simulink model "battery"  (R2021a)
settings: Solver=ode3  StartTime=0.0  StopTime=inf  FixedStep=T_est  RelTol=1e-3  EnableMultiTasking=on
values from neighbouring files (symbols this model uses):
  C1_array = [10000 10000 20775.14128 59367.58362 2271.12322 25499.34704 24626.77363 22758.69305 1470.76099 16269.06063 343.94923 166277.12244 ... (44 elements, 11x4)]    [ecmparams_vsc.mat]    (also in load_sim_data.m = [ecmparams(1:3,2)'; ecmparams(4:6,2)'; ecmparams(7:9,2)']; load_sim_data_v2.m = [ecmparams(1:3,2)'; ecmparams(4:6,2)'; ecmparams(7:9,2)'])
  C2_array = [5000 5000 3386.51997 1284.26954 733.57385 21.9068258 408.44714 1025.29527 23.88432 4732.43934 4.98786 7213.94612 ... (44 elements, 11x4)]    [ecmparams_vsc.mat]    (also in load_sim_data.m = [ecmparams(1:3,4)'; ecmparams(4:6,4)'; ecmparams(7:9,4)']; load_sim_data_v2.m = [ecmparams(1:3,4)'; ecmparams(4:6,4)'; ecmparams(7:9,4)'])
  cell_soc_init = initial_soc*ones(ns,nl,nc)    [load_sim_data.m]
  cell_temp = 25*ones(ns,nl,nc)    [load_sim_data.m]
  drive_profile = [0.003069801 0.003247245 0.003020715 0.003053892 0.002820143 0.003317081 0.003158873 0.002919445 0.002956375 0.002698265 0.002861501 0.002770798 ... (18750 elements, 1x18750)]    [drive_profile_ftp.mat]    (also in workspace.mat = [0 0 0 0 0 0 0 0 0 0 0 0 ... (521 elements, 1x521)]; workspace_2rc.mat; workspace_comparison.mat)
  drive_profile_index = [1 2 3 4 5 6 7 8 9 10 11 12 ... (18750 elements, 1x18750)]    [drive_profile_ftp.mat]    (also in load_sim_data_v2.m = drive_profile_index - 1; workspace.mat = [0 0.115384615385 0.230769230769 0.346153846154 0.4615384615; workspace_2rc.mat; workspace_comparison.mat)
  initial_soc = interp1(voc_soc_lut, voc_soc_lut_index, initial_vterm)    [load_sim_data.m]    (also in load_sim_data_v2.m)
  initial_temp = 25    [load_sim_data.m]    (also in load_sim_data_v2.m)
  nc = 1    [load_sim_data.m]
  nl = 1    [load_sim_data.m]
  nm = 1    [load_sim_data.m]
  ns = 1    [load_sim_data.m]
  Q_total = 236.8    [load_sim_data.m]    (also in load_sim_data_v2.m = 350; workspace.mat = 44; workspace_2rc.mat = 44; workspace_comparison.mat = 44)
  R1 = interp2(temp_array, voc_array, R1_array, initial_temp, initial_voc)    [load_sim_data.m]    (also in load_sim_data_v2.m; workspace.mat = 0.00033425; workspace_2rc.mat = 0.0001483; workspace_comparison.mat = 0.0001483)
  R1_array = [0.001 0.001 0.00171 0.00621 0.00621 0.00495 0.00657 0.00419 0.01404 0.0095 0.00356 0.01783 ... (44 elements, 11x4)]    [ecmparams_vsc.mat]    (also in load_sim_data.m = [ecmparams(1:3,3)'; ecmparams(4:6,3)'; ecmparams(7:9,3)']; load_sim_data_v2.m = [ecmparams(1:3,3)'; ecmparams(4:6,3)'; ecmparams(7:9,3)'])
  R2 = interp2(temp_array, voc_array, R2_array, initial_temp, initial_voc)    [load_sim_data.m]    (also in load_sim_data_v2.m; workspace.mat = 0.000915125; workspace_2rc.mat = 0.0001594; workspace_comparison.mat = 0.0001594)
  R2_array = [0.001 0.001 0.00067 0.01044 0.00794 0.01181 0.0098 0.00694 0.00323 0.00236 0.02009 0.00195 ... (44 elements, 11x4)]    [ecmparams_vsc.mat]    (also in load_sim_data.m = [ecmparams(1:3,5)'; ecmparams(4:6,5)'; ecmparams(7:9,5)']; load_sim_data_v2.m = [ecmparams(1:3,5)'; ecmparams(4:6,5)'; ecmparams(7:9,5)'])
  Ri = interp2(temp_array, voc_array, Ri_array, initial_temp, initial_voc)    [load_sim_data.m]    (also in load_sim_data_v2.m; workspace.mat = 0.000736040625; workspace_2rc.mat = 0.0007932; workspace_comparison.mat = 0.0007932)
  Ri_array = [0.001 0.001 0.00089 0.02157 0.01286 0.00303 0.0054 0.0079 0.00204 0.01221 0.00632 0.00315 ... (44 elements, 11x4)]    [ecmparams_vsc.mat]    (also in load_sim_data.m = [ecmparams(1:3,1)'; ecmparams(4:6,1)'; ecmparams(7:9,1)']; load_sim_data_v2.m = [ecmparams(1:3,1)'; ecmparams(4:6,1)'; ecmparams(7:9,1)'])
  sim_time = drive_profile_index(end)    [load_sim_data.m]    (also in load_sim_data_v2.m)
  temp_array = [15 25 35]    [load_sim_data.m]    (also in load_sim_data_v2.m)
  voc_array = [3 3.6 4.2]    [load_sim_data.m]    (also in load_sim_data_v2.m)
  voc_soc_lut = [3.07420931 3.44278771 3.51037487 3.58546258 3.63776945 3.68066188 3.73931818 3.84140797 3.94332291 4.0535654 4.18301283]    [emf_curve_single.mat]    (also in workspace.mat = [2.9985 3.0047 3.1504 3.2397 3.3026 3.3438 3.3699 3.3878 3.4; workspace_2rc.mat = [2.9985 3.0047 3.1504 3.2397 3.3026 3.3438 3.3699 3.3878 3.4; workspace_comparison.mat = [2.9985 3.0047 3.1504 3.2397 3.3026 3.3438 3.3699 3.3878 3.4)
  voc_soc_lut_index = [0 10 20 30 40 50 60 70 80 90 100]    [emf_curve_single.mat]    (also in workspace.mat = [0 1.6393442623 3.27868852459 4.91803278689 6.55737704918 8.; workspace_2rc.mat = [0 1.6393442623 3.27868852459 4.91803278689 6.55737704918 8.; workspace_comparison.mat = [0 1.6393442623 3.27868852459 4.91803278689 6.55737704918 8.)
undefined symbols (not defined in the file or in its folder): cell_c1_init, cell_c2_init, cell_r0_init, cell_r1_init, cell_r2_init
libraries: fl_lib x17, nesl_utility x11
settings Model: Creator=OTG00077  LastModifiedBy=avramkachura
settings SolverCC: AlgebraicLoopSolver=TrustRegion
settings DataIOCC: LimitDataPoints=on  SaveFormat=Array  ReturnWorkspaceOutputs=off
settings OptimizationCC: LifeSpan=inf
settings DebuggingCC: SolverPrmCheckMsg=warning  SFUnexpectedBacktrackingDiag=warning  SFNoUnconditionalDefaultTransitionDiag=warning  SFExecutionAtInitializationDiag=none  SFMachineParentedDataDiag=warning  ArithmeticOperatorsInVariantConditions=warning
settings HardwareCC: ProdBitPerPointer=32  ProdBitPerSizeT=32  ProdBitPerPtrDiffT=32  ProdLargestAtomicFloat=None  ProdIntDivRoundTo=Undefined  ProdEndianess=Unspecified  ProdWordSize=32  ProdHWDeviceType=32-bit Generic
settings ModelReferenceCC: PropagateSignalLabelsOutOfModel=off
settings SFSimCC: SimUseLocalCustomCode=off  CustomCodeUndefinedFunction=UseInterfaceOnly
settings RTWCC: RTWUseLocalCustomCode=off
settings CodeAppCC: StateflowObjectComments=on
settings GRTTargetCC: TargetLangStandard=C89/C90 (ANSI)
settings ConfigComp: CovMetricSettings=dw  CovSaveCumulativeToWorkspaceVar=on  CovSaveSingleToWorkspaceVar=on  CovExternalEMLEnable=off  CovSFcnEnable=off
settings SimscapeCC: SimscapeNormalizeSystem=off

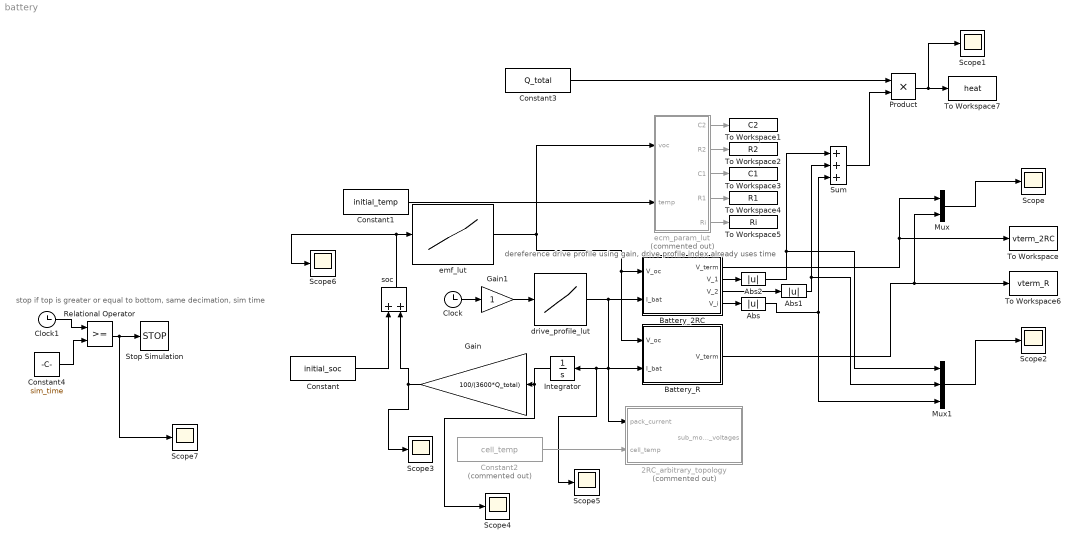
== system battery ==
  note: stop if top is greater or equal to bottom, same decimation, sim time
  note: dereference drive profile using gain, drive profile index already uses time
  2RC_arbitrary_topology : Subsystem  Commented=on
  Abs : Abs
  Abs1 : Abs
  Abs2 : Abs
  Battery_2RC : Subsystem
  Battery_R : Subsystem
  Clock : Clock
      settings: Decimation=100
  Clock1 : Clock
      settings: Decimation=100
  Constant : Constant  Value=initial_soc
  Constant1 : Constant  Value=initial_temp
  Constant2 : Constant  Commented=on  Value=cell_temp
  Constant3 : Constant  Value=Q_total
  Constant4 : Constant  Value=sim_time
  Gain : Gain  Gain=100/(3600*Q_total)
  Gain1 : Gain
  Integrator : Integrator
  Mux : Mux  Inputs=2
  Mux1 : Mux  Inputs=3
  Product : Product
  Relational Operator : RelationalOperator  OutDataTypeStr=boolean  RndMeth=Simplest
  Scope{,1..7} (8 alike) : Scope
  Stop Simulation : Stop
  Sum : Sum  Inputs=+++
  To Workspace : ToWorkspace  VariableName=vterm_2RC  SampleTime=-1
      settings: Decimation=100
  To Workspace1 : ToWorkspace  VariableName=C2  SampleTime=-1
      settings: MaxDataPoints=1  Decimation=100
  To Workspace2 : ToWorkspace  VariableName=R2  SampleTime=-1
      settings: MaxDataPoints=1  Decimation=100
  To Workspace3 : ToWorkspace  VariableName=C1  SampleTime=-1
      settings: MaxDataPoints=1  Decimation=100
  To Workspace4 : ToWorkspace  VariableName=R1  SampleTime=-1
      settings: MaxDataPoints=1  Decimation=100
  To Workspace5 : ToWorkspace  VariableName=Ri  SampleTime=-1
      settings: MaxDataPoints=1  Decimation=100
  To Workspace6 : ToWorkspace  VariableName=vterm_R  SampleTime=-1
      settings: Decimation=100
  To Workspace7 : ToWorkspace  VariableName=heat  SampleTime=-1
      settings: Decimation=100
  drive_profile_lut : Lookup_n-D  NumberOfTableDimensions=1  BreakpointsForDimension1=drive_profile_index  Table=drive_profile  InternalRulePriority=Speed  RndMeth=Simplest  InputSameDT=on
  "ecm_param_lut " : Subsystem  Commented=on
  emf_lut : Lookup_n-D  NumberOfTableDimensions=1  BreakpointsForDimension1=voc_soc_lut_index  Table=voc_soc_lut  InternalRulePriority=Speed  RndMeth=Simplest  InputSameDT=on
  soc : Sum
  wires:
  Integrator/1 -> Scope4/1, Gain/1
  Gain/1 -> Scope3/1, soc/2
  soc/1 -> Scope6/1, emf_lut/1
  Constant/1 -> soc/1
  emf_lut/1 -> "ecm_param_lut "/1(voc), Battery_R/1(V_oc), Battery_2RC/1(V_oc)
  drive_profile_lut/1 -> Battery_2RC/2(I_bat), Scope5/1, Integrator/1, 2RC_arbitrary_topology/1(pack_current), Battery_R/2(I_bat)
  Battery_2RC/1(V_term) -> Mux/1, To Workspace/1
  Clock/1 -> Gain1/1
  Gain1/1 -> drive_profile_lut/1
  Mux/1 -> Scope/1
  Battery_R/1(V_term) -> Mux/2, To Workspace6/1
  "ecm_param_lut "/1(C2) -> To Workspace1/1
  "ecm_param_lut "/2(R2) -> To Workspace2/1
  "ecm_param_lut "/5(Ri) -> To Workspace5/1
  "ecm_param_lut "/4(R1) -> To Workspace4/1
  "ecm_param_lut "/3(C1) -> To Workspace3/1
  Constant1/1 -> "ecm_param_lut "/2(temp)
  Constant2/1 -> 2RC_arbitrary_topology/2(cell_temp)
  Product/1 -> Scope1/1, To Workspace7/1
  Sum/1 -> Product/2
  Constant3/1 -> Product/1
  Battery_2RC/4(V_i) -> Abs/1
  Battery_2RC/3(V_2) -> Abs1/1
  Battery_2RC/2(V_1) -> Abs2/1
  Abs2/1 -> Mux1/1, Sum/1
  Abs1/1 -> Mux1/2, Sum/2
  Abs/1 -> Sum/3, Mux1/3
  Mux1/1 -> Scope2/1
  Relational Operator/1 -> Scope7/1, Stop Simulation/1
  Constant4/1 -> Relational Operator/2
  Clock1/1 -> Relational Operator/1

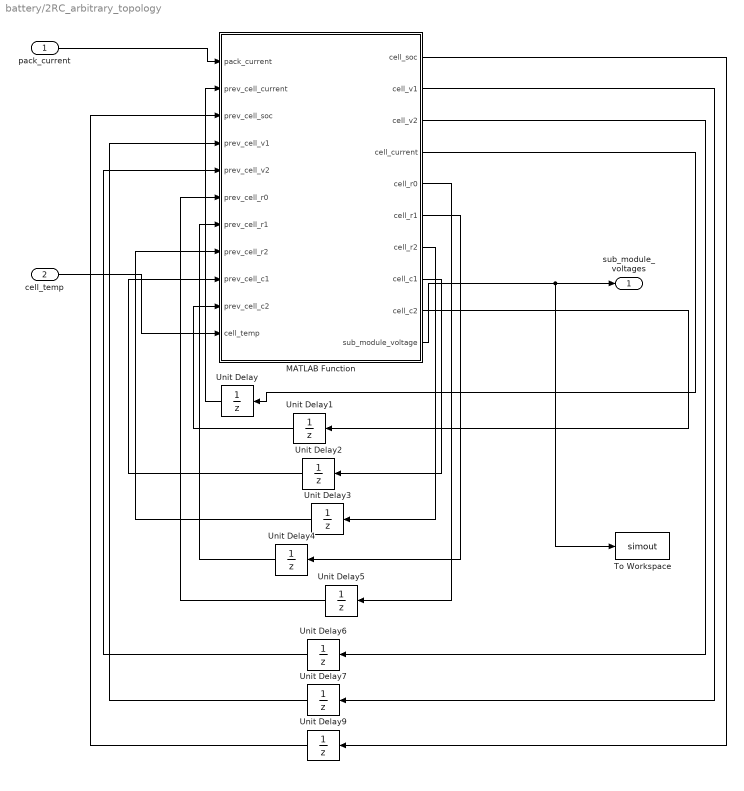
== system battery/2RC_arbitrary_topology ==
  pack_current : Inport
  cell_temp : Inport  Port=2
  MATLAB Function : MATLAB Function  TreatAsAtomicUnit=on
  To Workspace : ToWorkspace  VariableName=simout  SaveFormat=Timeseries  SampleTime=-1
  Unit Delay : UnitDelay  SampleTime=-1  HasFrameUpgradeWarning=on
  Unit Delay1 : UnitDelay  InitialCondition=cell_c2_init  SampleTime=-1  HasFrameUpgradeWarning=on
  Unit Delay2 : UnitDelay  InitialCondition=cell_c1_init  SampleTime=-1  HasFrameUpgradeWarning=on
  Unit Delay3 : UnitDelay  InitialCondition=cell_r2_init  SampleTime=-1  HasFrameUpgradeWarning=on
  Unit Delay4 : UnitDelay  InitialCondition=cell_r1_init  SampleTime=-1  HasFrameUpgradeWarning=on
  Unit Delay5 : UnitDelay  InitialCondition=cell_r0_init  SampleTime=-1  HasFrameUpgradeWarning=on
  Unit Delay6 : UnitDelay  SampleTime=-1  HasFrameUpgradeWarning=on
  Unit Delay7 : UnitDelay  SampleTime=-1  HasFrameUpgradeWarning=on
  Unit Delay9 : UnitDelay  InitialCondition=cell_soc_init  SampleTime=-1  HasFrameUpgradeWarning=on
  sub_module_voltages : Outport  VectorParamsAs1DForOutWhenUnconnected=off
  wires:
  pack_current/1 -> MATLAB Function/1(pack_current)
  cell_temp/1 -> MATLAB Function/11(cell_temp)
  MATLAB Function/10(sub_module_voltage) -> To Workspace/1, sub_module_voltages/1
  MATLAB Function/9(cell_c2) -> Unit Delay1/1
  Unit Delay1/1 -> MATLAB Function/10(prev_cell_c2)
  MATLAB Function/8(cell_c1) -> Unit Delay2/1
  Unit Delay2/1 -> MATLAB Function/9(prev_cell_c1)
  MATLAB Function/7(cell_r2) -> Unit Delay3/1
  Unit Delay3/1 -> MATLAB Function/8(prev_cell_r2)
  MATLAB Function/6(cell_r1) -> Unit Delay4/1
  Unit Delay4/1 -> MATLAB Function/7(prev_cell_r1)
  MATLAB Function/5(cell_r0) -> Unit Delay5/1
  Unit Delay5/1 -> MATLAB Function/6(prev_cell_r0)
  MATLAB Function/3(cell_v2) -> Unit Delay6/1
  Unit Delay6/1 -> MATLAB Function/5(prev_cell_v2)
  MATLAB Function/2(cell_v1) -> Unit Delay7/1
  Unit Delay7/1 -> MATLAB Function/4(prev_cell_v1)
  Unit Delay9/1 -> MATLAB Function/3(prev_cell_soc)
  MATLAB Function/4(cell_current) -> Unit Delay/1
  Unit Delay/1 -> MATLAB Function/2(prev_cell_current)
  MATLAB Function/1(cell_soc) -> Unit Delay9/1

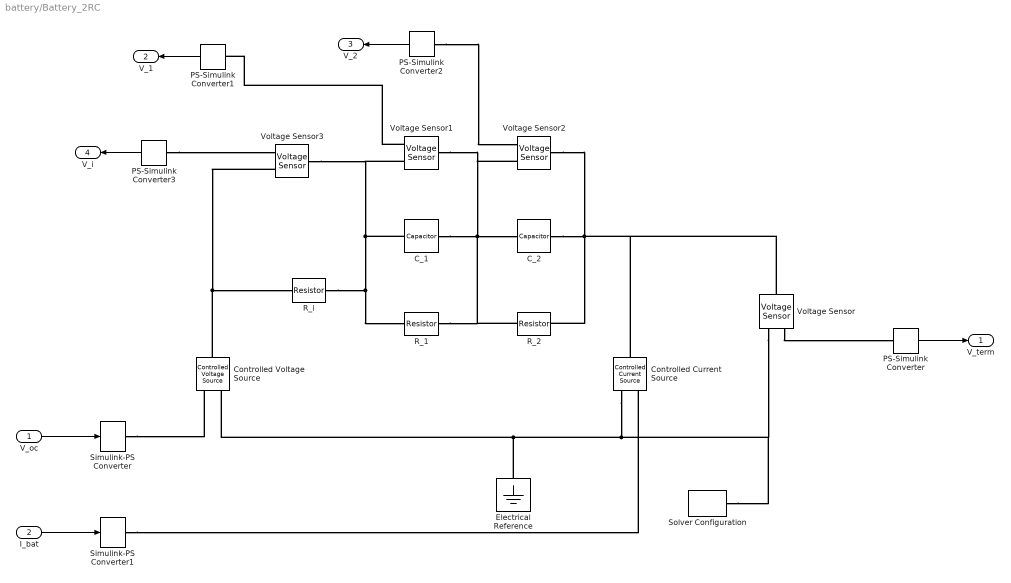
== system battery/Battery_2RC ==
  V_oc : Inport
  I_bat : Inport  Port=2
  C_1 : fl_lib/Electrical/Electrical Elements/Capacitor  c=C1 F  r=0 Ohm  g=0 1/Ohm  i_specify=off  i_priority=High  i=0 A  i_nominal_specify=off  i_nominal_unit=A  i_nominal_value=1  v_specify=off  v_priority=High  v=0 V  v_nominal_specify=off  v_nominal_unit=V  v_nominal_value=1  vc_specify=off  vc_priority=High  vc=0 V  vc_nominal_specify=off  vc_nominal_unit=V  vc_nominal_value=1
  C_2 : fl_lib/Electrical/Electrical Elements/Capacitor  c=C2 F  r=0 Ohm  g=0 1/Ohm  i_specify=off  i_priority=High  i=0 A  i_nominal_specify=off  i_nominal_unit=A  i_nominal_value=1  v_specify=off  v_priority=High  v=0 V  v_nominal_specify=off  v_nominal_unit=V  v_nominal_value=1  vc_specify=off  vc_priority=High  vc=0 V  vc_nominal_specify=off  vc_nominal_unit=V  vc_nominal_value=1
  Controlled Current Source : fl_lib/Electrical/Electrical Sources/Controlled Current Source
  Controlled Voltage Source : fl_lib/Electrical/Electrical Sources/Controlled Voltage Source
  Electrical Reference : fl_lib/Electrical/Electrical Elements/Electrical Reference
  PS-Simulink Converter{,1..3} (4 alike) : nesl_utility/PS-Simulink Converter  PhysicalDomain=network_engine_domain  SubClassName=ps_output  LeftPortType=input  RightPortType=output  PseudoPeriodic=off  Frequencies=[]  Unit=1  AffineConversion=off
      settings: SourceProductBaseCode=PW,SS
  R_1 : fl_lib/Electrical/Electrical Elements/Resistor  R=R1 Ohm  i_specify=off  i_priority=High  i=0 A  i_nominal_specify=off  i_nominal_unit=A  i_nominal_value=1  v_specify=off  v_priority=High  v=0 V  v_nominal_specify=off  v_nominal_unit=V  v_nominal_value=1
  R_2 : fl_lib/Electrical/Electrical Elements/Resistor  R=R2 Ohm  i_specify=off  i_priority=High  i=0 A  i_nominal_specify=off  i_nominal_unit=A  i_nominal_value=1  v_specify=off  v_priority=High  v=0 V  v_nominal_specify=off  v_nominal_unit=V  v_nominal_value=1
  R_i : fl_lib/Electrical/Electrical Elements/Resistor  R=Ri Ohm  i_specify=off  i_priority=High  i=0 A  i_nominal_specify=off  i_nominal_unit=A  i_nominal_value=1  v_specify=off  v_priority=High  v=0 V  v_nominal_specify=off  v_nominal_unit=V  v_nominal_value=1
  Simulink-PS Converter : nesl_utility/Simulink-PS Converter  PhysicalDomain=network_engine_domain  SubClassName=ps_input  LeftPortType=input  RightPortType=output  PseudoPeriodic=off  Frequencies=[]  NoiseDistribution=none  NoiseParameters=[]  Unit=1  AffineConversion=off  FilteringAndDerivatives=zero  SimscapeFilterOrder=1  InputFilterTimeConstant=0.001  UdotUserProvided=1
      settings: SourceProductBaseCode=PW,SS
  Simulink-PS Converter1 : nesl_utility/Simulink-PS Converter  PhysicalDomain=network_engine_domain  SubClassName=ps_input  LeftPortType=input  RightPortType=output  PseudoPeriodic=off  Frequencies=[]  NoiseDistribution=none  NoiseParameters=[]  Unit=1  AffineConversion=off  FilteringAndDerivatives=zero  SimscapeFilterOrder=1  InputFilterTimeConstant=0.001  UdotUserProvided=1
      settings: SourceProductBaseCode=PW,SS
  Solver Configuration : nesl_utility/Solver Configuration  PhysicalDomain=network_engine_domain  SubClassName=solver  LeftPortType=input  RightPortType=generic  Tones=[]  Harmonics=[]  SimulateNoise=off  Profile=off  UseLocalSampling=off  EnableSwitchedLinearOptims=on  FrequencyDomain=off  UseCCode=off  RelTol=0.001  AbsTol=1e-06  MinStep=1e-09  ToWorkspace=off  RevertToSquareIcSolve=off  NumHomotopyIterations=100  PhasorMode=off  PhasorModeNumHarmonics=1  DoDC=off  ResidualTolerance=1e-09  UseLocalSolver=off  LocalSolverChoice=NE_BACKWARD_EULER_ADVANCER  LocalSolverSampleTime=0.001  DoFixedCost=off  MaxNonlinIter=3  MaxModeIter=2  ComputeImpulses=off  ImpulseIterations=2  LinearAlgebra=Sparse  EquationFormulation=NE_TIME_EF  DelaysMemoryBudget=1024  AutomaticFiltering=on  FilteringTimeConstant=0.001  PartitionStorageMethod=AS_NEEDED  PartitionMemoryBudget=1024  PartitionMethod=FAST
      settings: SourceProductBaseCode=PW,SS
  Voltage Sensor{,1..3} (4 alike) : fl_lib/Electrical/Electrical Sensors/Voltage Sensor
  V_term : Outport  VectorParamsAs1DForOutWhenUnconnected=off
  V_1 : Outport  Port=2  VectorParamsAs1DForOutWhenUnconnected=off
  V_2 : Outport  Port=3  VectorParamsAs1DForOutWhenUnconnected=off
  V_i : Outport  Port=4  VectorParamsAs1DForOutWhenUnconnected=off
  wires:
  V_oc/1 -> Simulink-PS Converter/1
  PS-Simulink Converter/1 -> V_term/1
  I_bat/1 -> Simulink-PS Converter1/1
  PS-Simulink Converter1/1 -> V_1/1
  PS-Simulink Converter2/1 -> V_2/1
  PS-Simulink Converter3/1 -> V_i/1
  connections:
  R_i/RConn1 -- Voltage Sensor3/LConn1 -- Voltage Sensor1/RConn2 -- C_1/LConn1 -- R_1/LConn1
  C_1/RConn1 -- Voltage Sensor2/RConn2 -- Voltage Sensor1/LConn1 -- R_2/LConn1 -- R_1/RConn1 -- C_2/LConn1
  C_2/RConn1 -- Voltage Sensor2/LConn1 -- R_2/RConn1 -- Controlled Current Source/LConn1 -- Voltage Sensor/LConn1
  Controlled Voltage Source/LConn1 -- Voltage Sensor3/RConn2 -- R_i/LConn1
  Simulink-PS Converter/RConn1 -- Controlled Voltage Source/RConn1
  Voltage Sensor/RConn1 -- PS-Simulink Converter/LConn1
  Controlled Current Source/RConn2 -- Solver Configuration/RConn1 -- Voltage Sensor/RConn2 -- Electrical Reference/LConn1 -- Controlled Voltage Source/RConn2
  Simulink-PS Converter1/RConn1 -- Controlled Current Source/RConn1
  Voltage Sensor1/RConn1 -- PS-Simulink Converter1/LConn1
  PS-Simulink Converter2/LConn1 -- Voltage Sensor2/RConn1
  PS-Simulink Converter3/LConn1 -- Voltage Sensor3/RConn1

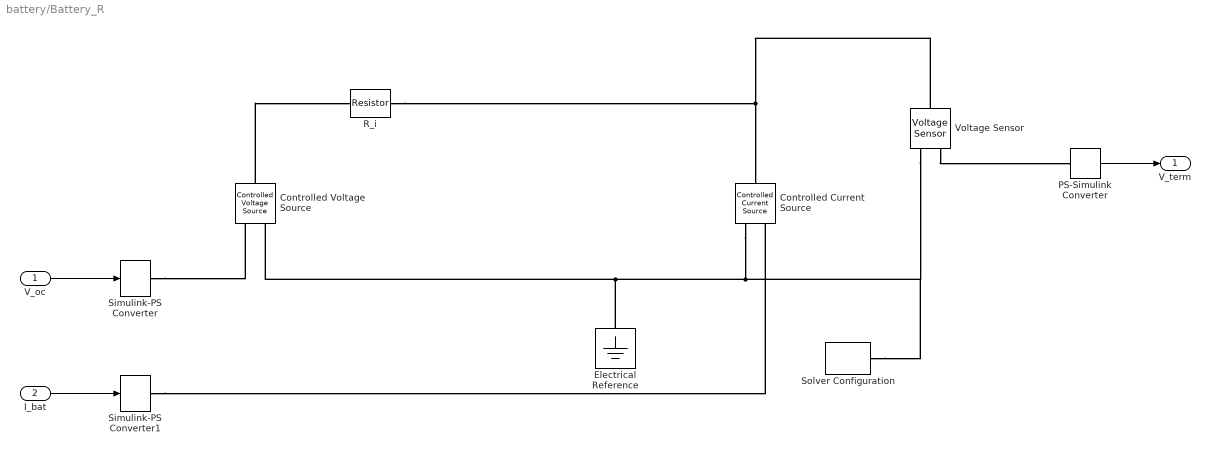
== system battery/Battery_R ==
  V_oc : Inport
  I_bat : Inport  Port=2
  Controlled Current Source : fl_lib/Electrical/Electrical Sources/Controlled Current Source
  Controlled Voltage Source : fl_lib/Electrical/Electrical Sources/Controlled Voltage Source
  Electrical Reference : fl_lib/Electrical/Electrical Elements/Electrical Reference
  PS-Simulink Converter : nesl_utility/PS-Simulink Converter  PhysicalDomain=network_engine_domain  SubClassName=ps_output  LeftPortType=input  RightPortType=output  PseudoPeriodic=off  Frequencies=[]  Unit=1  AffineConversion=off
      settings: SourceProductBaseCode=PW,SS
  R_i : fl_lib/Electrical/Electrical Elements/Resistor  R=Ri+R1+R2 Ohm  i_specify=off  i_priority=High  i=0 A  i_nominal_specify=off  i_nominal_unit=A  i_nominal_value=1  v_specify=off  v_priority=High  v=0 V  v_nominal_specify=off  v_nominal_unit=V  v_nominal_value=1
  Simulink-PS Converter : nesl_utility/Simulink-PS Converter  PhysicalDomain=network_engine_domain  SubClassName=ps_input  LeftPortType=input  RightPortType=output  PseudoPeriodic=off  Frequencies=[]  NoiseDistribution=none  NoiseParameters=[]  Unit=1  AffineConversion=off  FilteringAndDerivatives=zero  SimscapeFilterOrder=1  InputFilterTimeConstant=0.001  UdotUserProvided=1
      settings: SourceProductBaseCode=PW,SS
  Simulink-PS Converter1 : nesl_utility/Simulink-PS Converter  PhysicalDomain=network_engine_domain  SubClassName=ps_input  LeftPortType=input  RightPortType=output  PseudoPeriodic=off  Frequencies=[]  NoiseDistribution=none  NoiseParameters=[]  Unit=1  AffineConversion=off  FilteringAndDerivatives=zero  SimscapeFilterOrder=1  InputFilterTimeConstant=0.001  UdotUserProvided=1
      settings: SourceProductBaseCode=PW,SS
  Solver Configuration : nesl_utility/Solver Configuration  PhysicalDomain=network_engine_domain  SubClassName=solver  LeftPortType=input  RightPortType=generic  Tones=[]  Harmonics=[]  SimulateNoise=off  Profile=off  UseLocalSampling=off  EnableSwitchedLinearOptims=on  FrequencyDomain=off  UseCCode=off  RelTol=0.001  AbsTol=1e-06  MinStep=1e-09  ToWorkspace=off  RevertToSquareIcSolve=off  NumHomotopyIterations=100  PhasorMode=off  PhasorModeNumHarmonics=1  DoDC=off  ResidualTolerance=1e-09  UseLocalSolver=off  LocalSolverChoice=NE_BACKWARD_EULER_ADVANCER  LocalSolverSampleTime=0.001  DoFixedCost=off  MaxNonlinIter=3  MaxModeIter=2  ComputeImpulses=off  ImpulseIterations=2  LinearAlgebra=Sparse  EquationFormulation=NE_TIME_EF  DelaysMemoryBudget=1024  AutomaticFiltering=on  FilteringTimeConstant=0.001  PartitionStorageMethod=AS_NEEDED  PartitionMemoryBudget=1024  PartitionMethod=FAST
      settings: SourceProductBaseCode=PW,SS
  Voltage Sensor : fl_lib/Electrical/Electrical Sensors/Voltage Sensor
  V_term : Outport  VectorParamsAs1DForOutWhenUnconnected=off
  wires:
  V_oc/1 -> Simulink-PS Converter/1
  PS-Simulink Converter/1 -> V_term/1
  I_bat/1 -> Simulink-PS Converter1/1
  connections:
  Voltage Sensor/LConn1 -- Controlled Current Source/LConn1 -- R_i/RConn1
  Controlled Voltage Source/LConn1 -- R_i/LConn1
  Simulink-PS Converter/RConn1 -- Controlled Voltage Source/RConn1
  Voltage Sensor/RConn1 -- PS-Simulink Converter/LConn1
  Controlled Current Source/RConn2 -- Solver Configuration/RConn1 -- Voltage Sensor/RConn2 -- Electrical Reference/LConn1 -- Controlled Voltage Source/RConn2
  Simulink-PS Converter1/RConn1 -- Controlled Current Source/RConn1

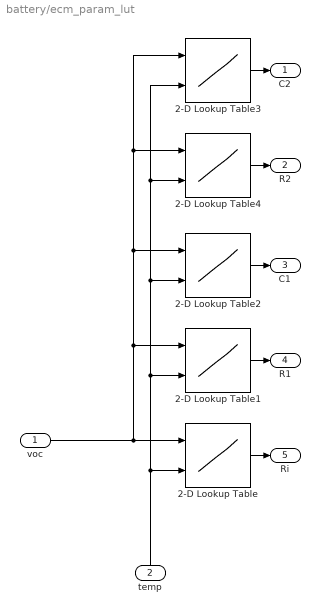
== system battery/ecm_param_lut  ==
  voc : Inport
  temp : Inport  Port=2
  2-D Lookup Table : Lookup_n-D  BreakpointsForDimension1=voc_array  BreakpointsForDimension2=temp_array  Table=Ri_array  ExtrapMethod=Clip  UseLastTableValue=on  InternalRulePriority=Speed  RndMeth=Simplest  InputSameDT=on
      settings: InputPortMap=u0,u1
  2-D Lookup Table1 : Lookup_n-D  BreakpointsForDimension1=voc_array  BreakpointsForDimension2=temp_array  Table=R1_array  ExtrapMethod=Clip  UseLastTableValue=on  InternalRulePriority=Speed  RndMeth=Simplest  InputSameDT=on
      settings: InputPortMap=u0,u1
  2-D Lookup Table2 : Lookup_n-D  BreakpointsForDimension1=voc_array  BreakpointsForDimension2=temp_array  Table=C1_array  ExtrapMethod=Clip  UseLastTableValue=on  InternalRulePriority=Speed  RndMeth=Simplest  InputSameDT=on
      settings: InputPortMap=u0,u1
  2-D Lookup Table3 : Lookup_n-D  BreakpointsForDimension1=voc_array  BreakpointsForDimension2=temp_array  Table=C2_array  ExtrapMethod=Clip  UseLastTableValue=on  InternalRulePriority=Speed  RndMeth=Simplest  InputSameDT=on
      settings: InputPortMap=u0,u1
  2-D Lookup Table4 : Lookup_n-D  BreakpointsForDimension1=voc_array  BreakpointsForDimension2=temp_array  Table=R2_array  ExtrapMethod=Clip  UseLastTableValue=on  InternalRulePriority=Speed  RndMeth=Simplest  InputSameDT=on
      settings: InputPortMap=u0,u1
  C2 : Outport  VectorParamsAs1DForOutWhenUnconnected=off
  R2 : Outport  Port=2  VectorParamsAs1DForOutWhenUnconnected=off
  C1 : Outport  Port=3  VectorParamsAs1DForOutWhenUnconnected=off
  R1 : Outport  Port=4  VectorParamsAs1DForOutWhenUnconnected=off
  Ri : Outport  Port=5  VectorParamsAs1DForOutWhenUnconnected=off
  wires:
  voc/1 -> 2-D Lookup Table1/1, 2-D Lookup Table2/1, 2-D Lookup Table4/1, 2-D Lookup Table3/1, 2-D Lookup Table/1
  2-D Lookup Table2/1 -> C1/1
  2-D Lookup Table4/1 -> R2/1
  2-D Lookup Table/1 -> Ri/1
  2-D Lookup Table1/1 -> R1/1
  2-D Lookup Table3/1 -> C2/1
  temp/1 -> 2-D Lookup Table3/2, 2-D Lookup Table4/2, 2-D Lookup Table2/2, 2-D Lookup Table1/2, 2-D Lookup Table/2

== matlab function battery/2RC_arbitrary_topology/MATLAB Function ==
  data: pack_current input double; cell_soc output double; prev_cell_current input double; prev_cell_soc input double; prev_cell_v1 input double; prev_cell_v2 input double; prev_cell_r0 input double; prev_cell_r1 input double; prev_cell_r2 input double; prev_cell_c1 input double; prev_cell_c2 input double; cell_v1 output double; cell_v2 output double; cell_temp input double; cell_current output double; cell_r0 output double; cell_r1 output double; cell_r2 output double; cell_c1 output double; cell_c2 output double; sub_module_voltage output double; nl parameter; nc parameter; ns parameter; nm parameter
function [cell_soc, cell_v1, cell_v2, cell_current, cell_r0, cell_r1, cell_r2, cell_c1, cell_c2, sub_module_voltage] = ...
    sm_calc(pack_current, prev_cell_current, prev_cell_soc, prev_cell_v1, prev_cell_v2, prev_cell_r0, ...
    prev_cell_r1, prev_cell_r2, prev_cell_c1, prev_cell_c2, cell_temp, ...
    nl, nc, ns, nm)

coder.extrinsic('evalin', 'assignin');

%% Import constants
% nl = 0;
% nl = evalin('base','nl');
% nc = 0;
% nc = evalin('base','nc');
% ns = 0;
% ns = evalin('base','ns');
% nm = 0;
% nm = evalin('base','nm');
R0_array = zeros(3,3);
R0_array = evalin('base','Ri_array');
R1_array = zeros(3,3);
R1_array = evalin('base','R1_array');
R2_array = zeros(3,3);
R2_array = evalin('base','R2_array');
C1_array = zeros(3,3);
C1_array = evalin('base','C1_array');
C2_array = zeros(3,3);
C2_array = evalin('base','C2_array');
Q_cell = 0;
Q_cell = evalin('base','Q_cell');
T_est = 0;
T_est = evalin('base','T_est');
temp_array = zeros(1,3);
temp_array = evalin('base','temp_array');
voc_array = zeros(1,3);
voc_array = evalin('base','voc_array');
voc_soc_lut = zeros(1,11);
voc_soc_lut = evalin('base','voc_soc_lut');
voc_soc_lut_index = zeros(1,11);
voc_soc_lut_index = evalin('base','voc_soc_lut_index');

%% Pack topology and local variables setup: Pack->String->Group->Link->Cell and also Module
cell_voc = zeros(ns,nl,nc);
cell_r0 = zeros(ns,nl,nc);
cell_r1 = zeros(ns,nl,nc);
cell_r2 = zeros(ns,nl,nc);
cell_c1 = zeros(ns,nl,nc);
cell_c2 = zeros(ns,nl,nc);
cell_soc = zeros(ns,nl,nc);
cell_v1 = zeros(ns,nl,nc);
cell_v2 = zeros(ns,nl,nc);
cell_current = zeros(ns,nl,nc);
sub_module_voltage = zeros(ns,1);
sum_vcell = zeros(ns,nl);
sum_r0 = zeros(ns,nl);
a = 0;
b = 0;

cell_temp=25*ones(ns,nl,nc);

%% Calculate current calculable states
for s = 1:ns
    for l = 1:nl
        for c = 1:nc
            cell_soc(s,l,c) = prev_cell_soc(s,l,c) + prev_cell_current(s,l,c)*T_est*100/(3600*Q_cell);
            cell_v1(s,l,c) = prev_cell_v1(s,l,c) + (T_est/prev_cell_c1(s,l,c))*(prev_cell_current(s,l,c)- ...
                prev_cell_v1(s,l,c)/prev_cell_r1(s,l,c));
            cell_v2(s,l,c) = prev_cell_v2(s,l,c) + (T_est/prev_cell_c2(s,l,c))*(prev_cell_current(s,l,c)- ...
                prev_cell_v2(s,l,c)/prev_cell_r2(s,l,c));
        end
    end
end

%% Calculate ECM parameters
for s = 1:ns
    for l = 1:nl
        for c = 1:nc
            cell_voc(s,l,c)=interp1(voc_soc_lut_index, voc_soc_lut, cell_soc(s,l,c));
            cell_r0(s,l,c)=s*interp2(temp_array, voc_array, R0_array, cell_temp(s,l,c), cell_voc(s,l,c));
            cell_c1(s,l,c)=interp2(temp_array, voc_array, C1_array, cell_temp(s,l,c), cell_voc(s,l,c));
            cell_r1(s,l,c)=interp2(temp_array, voc_array, R1_array, cell_temp(s,l,c), cell_voc(s,l,c));
            cell_c2(s,l,c)=interp2(temp_array, voc_array, C2_array, cell_temp(s,l,c), cell_voc(s,l,c));
            cell_r2(s,l,c)=interp2(temp_array, voc_array, R2_array, cell_temp(s,l,c), cell_voc(s,l,c));
        end
    end
end

%% Calculate cell currents

for s = 1:ns
    for l = 1:nl
        for c = 1:nc
            sum_vcell(s,l) = sum_vcell(s,l) + cell_v1(s,l,c) + cell_v2(s,l,c) + cell_voc(s,l,c);
            sum_r0(s,l) = sum_r0(s,l) + cell_r0(s,l,c);
        end
        a = a + sum_vcell(s,l)/sum_r0(s,l);
        b = b + 1/sum_r0(s,l);
    end
    sub_module_voltage(s) = (pack_current + a)/b;
    a = 0;
    b = 0;
end

for s = 1:ns
    for l = 1:nl
        for c = 1:nc
            cell_current(s,l,c) = (sub_module_voltage(s) - sum_vcell(s,l))/sum_r0(s,l);
        end
    end
end

end
